simulink subsystem "waterCoolingDuty"  (R2022b)
settings: Solver=VariableStepAuto  StartTime=0.0  StopTime=10.0  RelTol=1e-3
libraries: cooling_lib x3, Raptor_lib x3
settings Model: Creator=serga  LastModifiedBy=serga

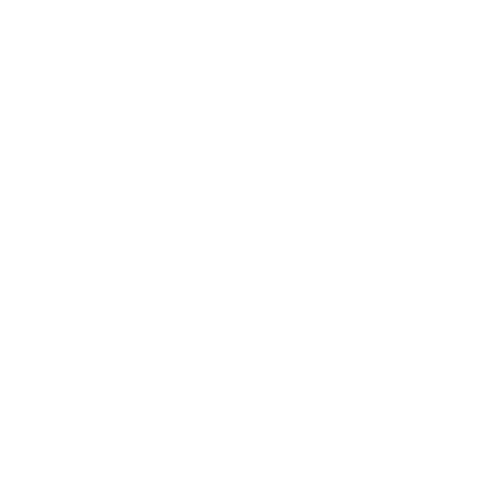
[thumbnail: Simulink's stored preview of the top-level diagram]
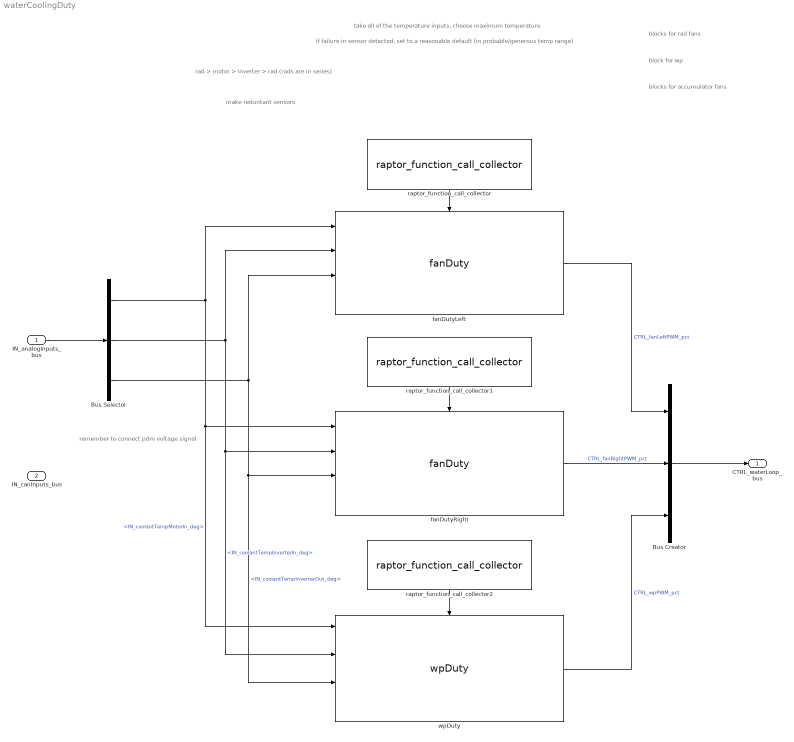
== system waterCoolingDuty ==
  note: remember to connect pdm voltage signal
  note: blocks for rad fans
  note: block for wp
  note: blocks for accumulator fans
  note: rad > motor > inverter > rad (rads are in series)
  note: make reduntant sensors
  note: take all of the temperature inputs, choose maximum temperature
  note: if failure in sensor detected, set to a reasonable default (in probable/generous temp range)
  IN_analogInputs_bus : Inport
  IN_canInputs_bus : Inport  Port=2
  Bus Creator : BusCreator  Inputs=3
  Bus Selector : BusSelector  OutputSignals=IN_coolantTemp_bus.IN_coolantTempMotorIn_bus.IN_coolantTempMotorIn_deg,IN_coolantTemp_bus.IN_coolantTempInverterIn_bus.IN_coolantTempInverterIn_deg,IN_coolantTemp_bus.IN_coolantTempInverterOut_bus.IN_coolantTempInverterOut_deg
  fanDutyLeft : cooling_lib/fanDuty  pos='Left'
  fanDutyRight : cooling_lib/fanDuty  pos='Right'
  raptor_function_call_collector : Raptor_lib/Triggers/raptor_function_call_collector  count=5
      settings: SourceProductName=Raptor
  raptor_function_call_collector1 : Raptor_lib/Triggers/raptor_function_call_collector  count=5
      settings: SourceProductName=Raptor
  raptor_function_call_collector2 : Raptor_lib/Triggers/raptor_function_call_collector  count=5
      settings: SourceProductName=Raptor
  wpDuty : cooling_lib/wpDuty  SystemSampleTime=-1  VariantActivationTime=update diagram  Latency=0  AutoFrameSizeCalculation=off
  CTRL_waterLoop_bus : Outport
  wires:
  raptor_function_call_collector/1 -> fanDutyLeft/Trigger
  IN_analogInputs_bus/1 -> Bus Selector/1
  Bus Selector/1 -> fanDutyRight/1, wpDuty/1, fanDutyLeft/1  "<IN_coolantTempMotorIn_deg>"
  Bus Selector/2 -> fanDutyRight/2, wpDuty/2, fanDutyLeft/2  "<IN_coolantTempInverterIn_deg>"
  Bus Selector/3 -> fanDutyRight/3, wpDuty/3, fanDutyLeft/3  "<IN_coolantTempInverterOut_deg>"
  raptor_function_call_collector1/1 -> fanDutyRight/Trigger
  fanDutyLeft/1 -> Bus Creator/1  "CTRL_fanLeftPWM_pct"
  fanDutyRight/1 -> Bus Creator/2  "CTRL_fanRightPWM_pct"
  Bus Creator/1 -> CTRL_waterLoop_bus/1
  raptor_function_call_collector2/1 -> wpDuty/Trigger
  wpDuty/1 -> Bus Creator/3  "CTRL_wpPWM_pct"
